simulink model "mymodel"  (R2017b)
settings: Solver=VariableStepAuto  StartTime=0.0  StopTime=20.0  RelTol=1e-3
values from neighbouring files (symbols this model uses):
  stepf = 0    [mass_spring_damper_script.m]    (also in mymodel_sim.m = 10)
  stepi = 2    [mass_spring_damper_script.m]    (also in mymodel_sim.m = 0)
  stept = 1    [mass_spring_damper_script.m]    (also in mymodel_sim.m)
  tau = 0.5    [mymodel_sim.m]
  x0 = 0    [mymodel_sim.m]
settings Model: Creator=Koh Kim Hai  LastModifiedBy=Koh Kim Hai
settings DataIOCC: TimeSaveName=mytime

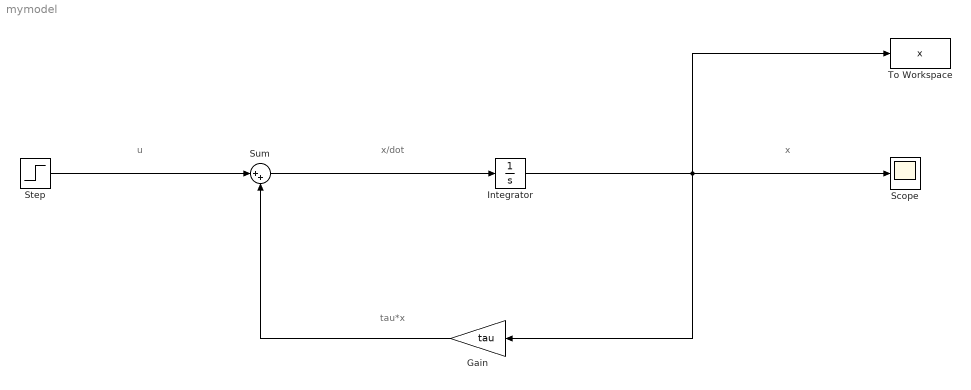
== system mymodel ==
  note: tau*x
  note: u
  note: x
  note: x/dot
  Gain : Gain  Gain=tau
  Integrator : Integrator  InitialCondition=x0
  Scope : Scope
  Step : Step  Time=stept  Before=stepi  After=stepf  SampleTime=0
  Sum : Sum  Inputs=|++
  To Workspace : ToWorkspace  VariableName=x  SampleTime=-1
  wires:
  Step/1 -> Sum/1
  Gain/1 -> Sum/2
  Sum/1 -> Integrator/1
  Integrator/1 -> Gain/1, To Workspace/1, Scope/1
